simulink model "dspg711amua"  (Simulink 5.0)
settings: Solver=FixedStepDiscrete  StartTime=0.0  StopTime=4.99  RelTol=1e-3
PreLoadFcn:
  | frmSize=256;[cleve,Fs]=wavread('speech_dft.wav');
undefined symbols (not defined in the file or in its folder): Fs, magnitude
libraries: dspquant2 x6, dspstat3 x2, dspbuff3 x2, dspsigattribs x1, simulink x1, dspmathops x1, dspsrcs4 x1
settings Model: Creator=mani  LastModifiedBy=mkhan  ExtModeAutoUpdateStatusClock=off  SignalLoggingName=logsOut  BooleanDataType=off  ZeroCrossControl=UseLocalSettings  TargetHWChar=2  TargetHWWordLengths=8,16,32,32  RTWMathFcnLibMatFile=iso_c_tmw.mat  RTWOptions="-aEnforceIntegerDowncast=1 -aFoldNonRolledExpr=1 -aInlineInvariantSignals=1 -aInlineParameters=0 -aLocalBlockOutputs=1 -aRollThreshold=5 -aRTWVerbose=1 -aForceParamTrailComments=0 -aGenerateComments=1 -aIgnoreCustomStorageClasses=1 -aIncHierarchyInIds=0 -aMaxRTWIdLen=31 -aShowEliminatedStatements=0 -aReadOnly=0 -aTargetFcnLib=\"iso_c_tmw.mat\" -aIncDataTypeInIds=0 -aPrefixModelToSubsysFcnNames=1 -aInlinedPrmAccess=\"Literals\" -aGenerateFullHeader=1 -aIsPILTarget=0 -aGenerateReport=0 -aLogVarNameModifier=\"rt_\" -aExtMode=0 -aExtModeStaticAlloc=0 -aExtModeTesting=0 -aExtModeStaticAllocSize=1000000 -aExtModeTransport=0"

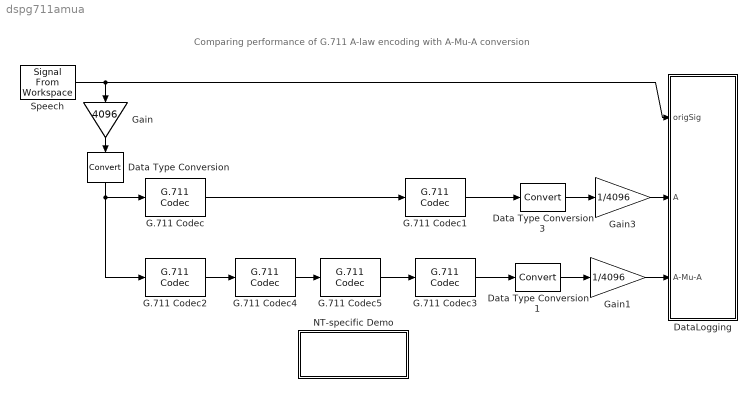
== system dspg711amua ==
  note: Comparing performance of G.711 A-law encoding with A-Mu-A conversion
  Data Type Conversion : DataTypeConversion  Orientation=down  OutDataTypeMode=int16  SaturateOnIntegerOverflow=on  RndMeth=Zero
  Data Type Conversion1 : DataTypeConversion  OutDataTypeMode=double  SaturateOnIntegerOverflow=on  RndMeth=Zero
  Data Type Conversion3 : DataTypeConversion  OutDataTypeMode=double  SaturateOnIntegerOverflow=on  RndMeth=Zero
  DataLogging : Subsystem
  G.711 Codec : dspquant2/G.711 Codec  mode=Encode PCM to A-law  errmode=Warning
  G.711 Codec1 : dspquant2/G.711 Codec  mode=Decode A-law to PCM  errmode=Warning
  G.711 Codec2 : dspquant2/G.711 Codec  mode=Encode PCM to A-law  errmode=Warning
  G.711 Codec3 : dspquant2/G.711 Codec  mode=Decode A-law to PCM  errmode=Warning
  G.711 Codec4 : dspquant2/G.711 Codec  mode=Convert A-law to mu-law  errmode=Warning
  G.711 Codec5 : dspquant2/G.711 Codec  mode=Convert mu-law to A-law  errmode=Warning
  Gain : Gain  Orientation=down  Gain=4096  SaturateOnIntegerOverflow=on
  Gain1 : Gain  Gain=1/4096  SaturateOnIntegerOverflow=on
  Gain3 : Gain  Gain=1/4096  SaturateOnIntegerOverflow=on
  NT-specific Demo : Subsystem
      settings: OpenFcn=dspg711amua_mic
      mask Type: NT-only Demo
      mask Display: disp('PC/Windows\nDemo')
  Speech : dspsrcs4/Signal From Workspace  X=cleve  Ts=1/Fs  nsamps=frmSize  OutputAfterFinalValue=Setting to zero
  wires:
  G.711 Codec3/1 -> Data Type Conversion1/1
  Gain/1 -> Data Type Conversion/1
  Data Type Conversion1/1 -> Gain1/1
  Gain1/1 -> DataLogging/3(A-Mu-A)
  Data Type Conversion/1 -> G.711 Codec/1, G.711 Codec2/1
  G.711 Codec1/1 -> Data Type Conversion3/1
  G.711 Codec/1 -> G.711 Codec1/1
  Data Type Conversion3/1 -> Gain3/1
  Gain3/1 -> DataLogging/2(A)
  Speech/1 -> Gain/1, DataLogging/1(origSig)
  G.711 Codec5/1 -> G.711 Codec3/1
  G.711 Codec4/1 -> G.711 Codec5/1
  G.711 Codec2/1 -> G.711 Codec4/1

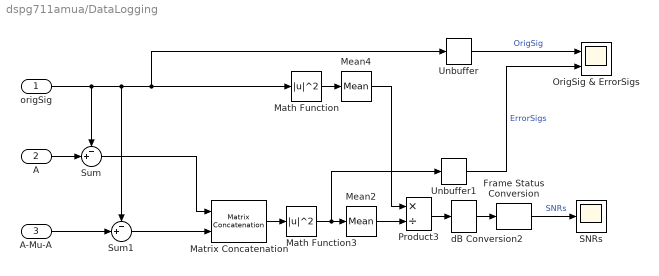
== system dspg711amua/DataLogging ==
  origSig : Inport
  A : Inport  Port=2
  A-Mu-A : Inport  Port=3
  Frame Status Conversion : dspsigattribs/Frame Status Conversion  growRefPort=off  outframe=Sample-based
  Math Function : Math  Operator=magnitude^2
  Math Function3 : Math  Operator=magnitude^2
  Matrix Concatenation : simulink/Math Operations/Matrix Concatenation  numInports=2  catMethod=Horizontal
  Mean2 : dspstat3/Mean  run=off  reset_popup=None
  Mean4 : dspstat3/Mean  run=off  reset_popup=None
  OrigSig & ErrorSigs : Scope  NumInputPorts=2
      settings: TimeRange=5  YMin=-1.2~0  YMax=1.2~0.00045  MaxDataPoints=80000
  Product3 : Product  Inputs=*/  SaturateOnIntegerOverflow=on  RndMeth=Zero  InputSameDT=on
  SNRs : Scope
      settings: TimeRange=5  YMin=0  YMax=50
  Sum : Sum  Inputs=-+|  SaturateOnIntegerOverflow=on  InputSameDT=on
  Sum1 : Sum  Inputs=-+|  SaturateOnIntegerOverflow=on  InputSameDT=on
  Unbuffer : dspbuff3/Unbuffer  ic=0
  Unbuffer1 : dspbuff3/Unbuffer  ic=0
  dB Conversion2 : dspmathops/dB Conversion  dBtype=dB  intype=Power  R=1  fuzz=on
  wires:
  Unbuffer1/1 -> OrigSig & ErrorSigs/2  "ErrorSigs"
  Unbuffer/1 -> OrigSig & ErrorSigs/1  "OrigSig"
  Frame Status Conversion/1 -> SNRs/1  "SNRs"
  dB Conversion2/1 -> Frame Status Conversion/1
  Product3/1 -> dB Conversion2/1
  Mean2/1 -> Product3/2
  Mean4/1 -> Product3/1
  Math Function3/1 -> Unbuffer1/1, Mean2/1
  Matrix Concatenation/1 -> Math Function3/1
  Sum1/1 -> Matrix Concatenation/2
  Sum/1 -> Matrix Concatenation/1
  Math Function/1 -> Mean4/1
  A-Mu-A/1 -> Sum1/2
  A/1 -> Sum/2
  origSig/1 -> Unbuffer/1, Math Function/1, Sum1/1, Sum/1

== system dspg711amua/NT-specific Demo ==
